simulink model "test_quad_mpc"  (R2020a)
settings: Solver=VariableStepAuto  StartTime=0.0  StopTime=10.0  RelTol=1e-3
settings Model: Creator=kekatos  LastModifiedBy=kekatos
settings SolverCC: ZeroCrossAlgorithm=Adaptive

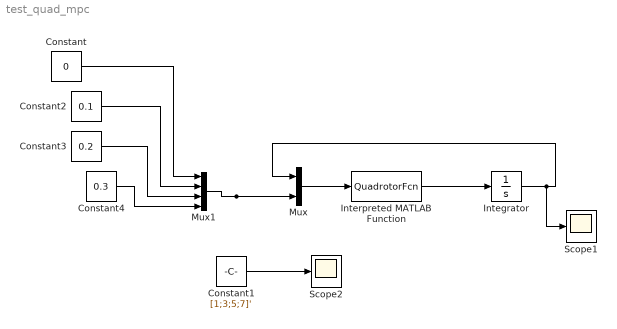
== system test_quad_mpc ==
  Constant : Constant  Value=0
  Constant1 : Constant  Value=[1;3;5;7]'  VectorParams1D=off
  Constant2 : Constant  Value=0.1
  Constant3 : Constant  Value=0.2
  Constant4 : Constant  Value=0.3
  Integrator : Integrator
  Interpreted MATLAB Function : MATLABFcn  MATLABFcn=QuadrotorFcn  OutputDimensions=12
  Mux : Mux  Inputs=2
  Mux1 : Mux
  Scope1 : Scope
  Scope2 : Scope
  wires:
  Interpreted MATLAB Function/1 -> Integrator/1
  Constant1/1 -> Scope2/1
  Mux/1 -> Interpreted MATLAB Function/1
  Integrator/1 -> Scope1/1, Mux/1
  Constant/1 -> Mux1/1
  Constant2/1 -> Mux1/2
  Constant3/1 -> Mux1/3
  Constant4/1 -> Mux1/4
  Mux1/1 -> Mux/2
